simulink model "TWIP_NL"  (R2025b)
settings: Solver=ode45  StartTime=0.0  StopTime=10  MaxStep=0.02  RelTol=1e-4  AbsTol=1e-6
values from neighbouring files (symbols this model uses):
  d1_ext = 0    [twip_params.m]
  d2_ext = 0    [twip_params.m]
  K_lqr = twip_p.K_lqr    [twip_params.m]
  p_bache = [twip_p.bache_pos; twip_p.bache_h; twip_p.bache_w]    [twip_params.m]
  p_phys = [twip_p.mB, twip_p.mW, twip_p.r,  twip_p.dw, twip_p.l,  twip_p.g,             twip_p.I1,  twip_p.I2,  twip_p.I3, twip_p.J,  twip_p.K]'    [twip_params.m]
  X0 = [0; 0.05; 0; 0.0; 0; 0]    [twip_params.m]
settings Model: Creator=crist  LastModifiedBy=crist

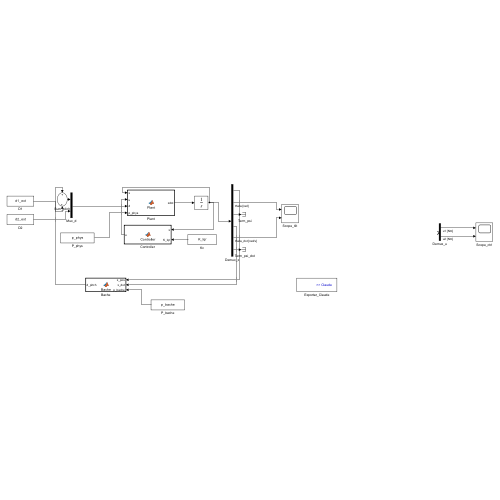
[thumbnail: Simulink's stored preview of the top-level diagram]
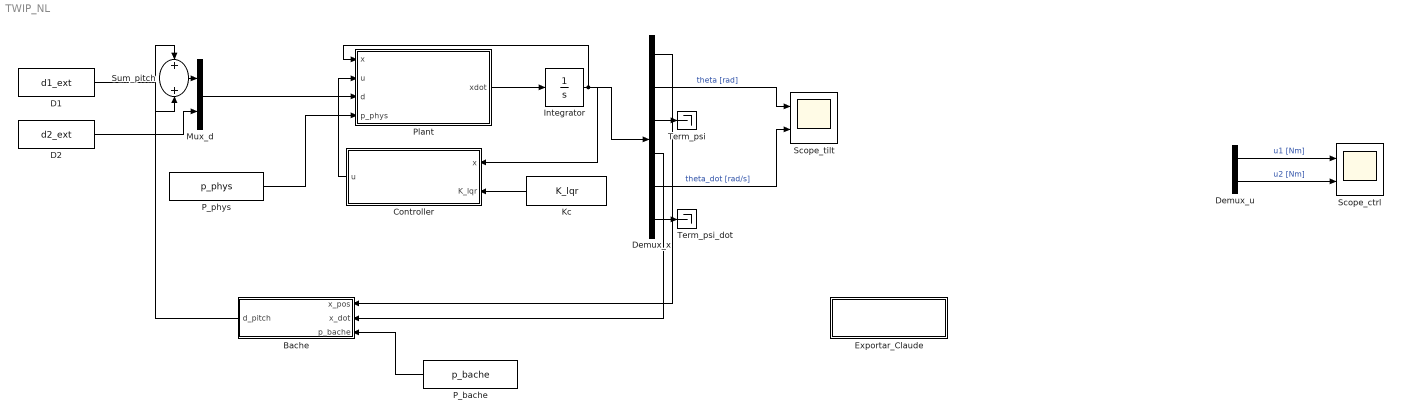
== system TWIP_NL ==
  Bache : MATLAB Function  TreatAsAtomicUnit=on
  Controller : MATLAB Function  TreatAsAtomicUnit=on
  D1 : Constant  Value=d1_ext
  D2 : Constant  Value=d2_ext
  Demux_u : Demux  Outputs=2
  Demux_x : Demux  Outputs=6
  Exportar_Claude : Subsystem
      settings: OpenFcn=addpath(fileparts(get_param(bdroot,'FileName'))); run('export_model_state');
      mask Display:
      | color('blue');
      | text(0.5,0.5,'>> Claude');
  Integrator : Integrator  InitialCondition=X0
  Kc : Constant  Value=K_lqr
  Mux_d : Mux  Inputs=2
  P_bache : Constant  Value=p_bache
  P_phys : Constant  Value=p_phys
  Plant : MATLAB Function  TreatAsAtomicUnit=on
  Scope_ctrl : Scope  NumInputPorts=2
      settings: Title=Torques de control
  Scope_tilt : Scope  NumInputPorts=2
      settings: Title=Cabeceo
  Sum_pitch : Sum
  Term_psi : Terminator
  Term_psi_dot : Terminator
  wires:
  Plant/1(xdot) -> Integrator/1
  Integrator/1 -> Plant/1(x), Demux_x/1, Controller/1(x)
  P_phys/1 -> Plant/4(p_phys)
  Kc/1 -> Controller/2(K_lqr)
  Controller/1(u) -> Plant/2(u)
  Bache/1(d_pitch) -> Sum_pitch/1
  D1/1 -> Sum_pitch/2
  Sum_pitch/1 -> Mux_d/1
  D2/1 -> Mux_d/2
  Mux_d/1 -> Plant/3(d)
  Demux_x/1 -> Bache/1(x_pos)
  Demux_x/4 -> Bache/2(x_dot)
  P_bache/1 -> Bache/3(p_bache)
  Demux_x/3 -> Term_psi/1
  Demux_x/6 -> Term_psi_dot/1
  Demux_x/2 -> Scope_tilt/1  "theta [rad]"
  Demux_x/5 -> Scope_tilt/2  "theta_dot [rad/s]"
  Demux_u/1 -> Scope_ctrl/1  "u1 [Nm]"
  Demux_u/2 -> Scope_ctrl/2  "u2 [Nm]"

== system TWIP_NL/Exportar_Claude ==

== matlab function TWIP_NL/Controller ==
  data: x input; u output; K_lqr input
function u = Controller(x, K_lqr)
u = twip_ctrl_lqr(x, K_lqr);
end

== matlab function TWIP_NL/Plant ==
  data: x input; u input; xdot output; d input; p_phys input
function xdot = Plant(x, u, d, p_phys)
xdot = twip_plant_fcn(x, u, d, p_phys);
end

== matlab function TWIP_NL/Bache ==
  data: x_pos input; d_pitch output; x_dot input; p_bache input
function d_pitch = Bache(x_pos, x_dot, p_bache)
d_pitch = twip_bache_fcn(x_pos, x_dot, p_bache);
end
